simulink library "tqd"  (R2021b)
settings: Solver=VariableStepAuto  StartTime=0.0  StopTime=10.0  RelTol=1e-3
undefined symbols (not defined in the file or in its folder): ATQD_APSDecReq_X_kph, ATQD_APSDecReq_Y_mps2, ATQD_APSDecReqCMD_X_kph, ATQD_APSDecReqTs_X_pct, ATQD_APSDecTimeGain_X_Deg, ATQD_APSDecTimeGain_Y_s, ATQD_APSReqLowSpd_X_Deg, ATQD_AutoHoldReleaseBPS_X_Deg, ATQD_AWDLoadTrqnsGain_X_kg, ATQD_AWDLoadTrqnsGain_Y_pct, ATQD_BOSEnBPSPosn_X_kph, ATQD_BOSMap_X_rpm, ATQD_BOSMap_Y_pct, ATQD_CreepBaseTqD_X_kph, ATQD_CreepBaseTqD_Y_Deg, ATQD_CreepBaseTqR_X_kph, ATQD_CreepBaseTqR_Y_Deg, ATQD_CreepBPSDisPosn_X_Deg, ATQD_CreepBPSDisPosnR_X_Deg, ATQD_CreepBPSEnPosn_X_Deg, ATQD_CreepBPSEnPosnR_X_Deg, ATQD_CreepDeltaTq_X_kph, ATQD_CreepIterm_X_kph, ATQD_CreepIterm_Y_kph, ATQD_CreepItermMaxLimit_X_pct, ATQD_CreepPreloadTime_X_kph, ATQD_CreepPreloadTq_X_kph, ATQD_CreepPreloadTq_Y_s, ATQD_CreepProtTq_X_Deg, ATQD_CreepPterm_X_kph, ATQD_CreepPterm_Y_kph, ATQD_ECOTqMapD_X_rpm, ATQD_ECOTqMapD_Y_pct, ATQD_EOPDTqMapDCon_X_rpm, ATQD_EOPDTqMapDCon_Y_Deg, ATQD_EstInitVehWeight_X_c, ATQD_LHMRollGenMapD_X_rpm, ATQD_LHMRollGenMapD_Y_rpm, ATQD_LHMTqMapD_X_rpm, ATQD_LHMTqMapD_Y_pct, ATQD_NL1TqMapD_X_rpm, ATQD_NL1TqMapD_Y_pct, ATQD_NOPDTqMapDCon_X_rpm, ATQD_NOPDTqMapDCon_Y_Deg, ATQD_NRMRrEDUSpRat_X_rpm, ATQD_NRMRrEDUSpRat_Y_Nm, ATQD_OPDHoldDownRelDelay_X_Deg, ATQD_OPDHoldEnSpd_X_Deg, ATQD_OPDHoldRelDetTime_X_Deg, ATQD_OPDHoldReleaseTq_X_Deg, ATQD_OrigPedTqLowLim_X_Deg, ATQD_OrigPedTqLowLim_Y_pct, ATQD_PedalMapClimbUpLim_X_rpm, ATQD_PedalMapClimbUpLim_Y_Deg, ATQD_PreLoadTq_X_s, ATQD_RollGenMapEL1_X_rpm, ATQD_RollGenMapEL1_Y_rpm, ATQD_SL1TqMapD_X_rpm, ATQD_SL1TqMapD_Y_pct, ATQD_SlideRegenTqGain_X_Gps ... (+491)
libraries: hcu_lib x83, simulink x73, tqr x1
(part 15 of 19)

== system tqd/TQD/TorqueDemand/TorqueModule/DriverWhlTqDem/PedalMapWhlTq/NoLHM/ShiftD/LUT_D_Normal ==
  VTQD_TqTargetShaftSpd_rpm : Inport
  VTQD_ActAPSPosn_pct : Inport  Port=2
  VTQD_RegenMode_enum : Inport  Port=3
  VVMC_EstSlope_Deg : Inport  Port=4
  VTQD_APSReqTimer_s : Inport  Port=5
  VTQD_LowIdleAccPedal_flg : Inport  Port=6
  VTQD_OPDHoldEnRel_flg : Inport  Port=7
  VTQD_OPDHoldActRelTq_Nm : Inport  Port=8
  VTQD_VehActSpd_kph : Inport  Port=9
  VTQD_SlopeUp_flg : Inport  Port=10
  Action Port : ActionPort  ActionPortLabel=elseif(u2 ~= 0)
  Constant : Constant  Value=ENUM_REGENLEVEL_LV1
  Constant1 : Constant  Value=ENUM_REGENLEVEL_LV2
  Constant2 : Constant  Value=ENUM_REGENLEVEL_LV3
  Constant3 : Constant  Value=ENUM_REGENLEVEL_LV4
  Constant4 : Constant  Value=ENUM_REGENLEVEL_LV5
  Constant5 : Constant  Value=ENUM_REGENLEVEL_OPD
  Equal{1..6} (6 alike) : RelationalOperator  Operator===  OutDataTypeStr=boolean  RndMeth=Simplest
  If : If  NumInputs=6  IfExpression=u1 ~= 0  ElseIfExpressions=u2 ~= 0, u3 ~= 0, u4 ~= 0, u5 ~= 0, u6~=0
  MTQD_NL1TqMapD_Z_Nm : Lookup_n-D  BreakpointsForDimension1=ATQD_NL1TqMapD_Y_pct  BreakpointsForDimension2=ATQD_NL1TqMapD_X_rpm  Table=MTQD_NL1TqMapD_Z_Nm  ExtrapMethod=Clip  InternalRulePriority=Speed  RndMeth=Simplest  InputSameDT=on
      settings: InputPortMap=u0,u1
  MTQD_NL2TqMapD_Z_Nm : Lookup_n-D  BreakpointsForDimension1=ATQD_NL1TqMapD_Y_pct  BreakpointsForDimension2=ATQD_NL1TqMapD_X_rpm  Table=MTQD_NL2TqMapD_Z_Nm  ExtrapMethod=Clip  InternalRulePriority=Speed  RndMeth=Simplest  InputSameDT=on
      settings: InputPortMap=u0,u1
  MTQD_NL3TqMapD_Z_Nm : Lookup_n-D  BreakpointsForDimension1=ATQD_NL1TqMapD_Y_pct  BreakpointsForDimension2=ATQD_NL1TqMapD_X_rpm  Table=MTQD_NL3TqMapD_Z_Nm  ExtrapMethod=Clip  InternalRulePriority=Speed  RndMeth=Simplest  InputSameDT=on
      settings: InputPortMap=u0,u1
  MTQD_NL4TqMapD_Z_Nm1 : Lookup_n-D  BreakpointsForDimension1=ATQD_NL1TqMapD_Y_pct  BreakpointsForDimension2=ATQD_NL1TqMapD_X_rpm  Table=MTQD_NL4TqMapD_Z_Nm  ExtrapMethod=Clip  InternalRulePriority=Speed  RndMeth=Simplest  InputSameDT=on
      settings: InputPortMap=u0,u1
  MTQD_NL5TqMapD_Z_Nm1 : Lookup_n-D  BreakpointsForDimension1=ATQD_NL1TqMapD_Y_pct  BreakpointsForDimension2=ATQD_NL1TqMapD_X_rpm  Table=MTQD_NL5TqMapD_Z_Nm  ExtrapMethod=Clip  InternalRulePriority=Speed  RndMeth=Simplest  InputSameDT=on
      settings: InputPortMap=u0,u1
  MTQD_NOPDTqMapDCon_Z_Nm : Lookup_n-D  BreakpointsForDimension1=ATQD_NOPDTqMapDCon_Y_Deg  BreakpointsForDimension2=ATQD_NOPDTqMapDCon_X_rpm  Table=MTQD_NOPDTqMapDCon_Z_Nm  ExtrapMethod=Clip  InternalRulePriority=Speed  RndMeth=Simplest  InputSameDT=on
      settings: InputPortMap=u0,u1
  MTQD_NOPDTqMapD_Z_Nm1 : Lookup_n-D  BreakpointsForDimension1=ATQD_NL1TqMapD_Y_pct  BreakpointsForDimension2=ATQD_NL1TqMapD_X_rpm  Table=MTQD_NOPDTqMapD_Z_Nm  ExtrapMethod=Clip  InternalRulePriority=Speed  RndMeth=Simplest  InputSameDT=on
      settings: InputPortMap=u0,u1
  Merge : Merge  Inputs=7
  NRM_Invalid_TqMap1 : Subsystem  TreatAsAtomicUnit=on
  NRM_Lv1_TqMap : Subsystem  TreatAsAtomicUnit=on
  NRM_Lv2_TqMap : Subsystem  TreatAsAtomicUnit=on
  NRM_Lv3_TqMap : Subsystem  TreatAsAtomicUnit=on
  NRM_Lv4_TqMap : Subsystem  TreatAsAtomicUnit=on
  NRM_Lv5_TqMap : Subsystem  TreatAsAtomicUnit=on
  NRM_OnePedal_TqMap : Subsystem  TreatAsAtomicUnit=on
  VTQD_WhlTqNRMD_Nm : Outport
  wires:
  Equal6/1 -> If/6
  [VTQD_RegenMode_enum] -> Equal6/1
  Constant5/1 -> Equal6/2
  Equal5/1 -> If/5
  [VTQD_RegenMode_enum] -> Equal5/1
  Constant4/1 -> Equal5/2
  Equal4/1 -> If/4
  [VTQD_RegenMode_enum] -> Equal4/1
  Constant3/1 -> Equal4/2
  [VTQD_RegenMode_enum] -> Equal3/1
  Constant2/1 -> Equal3/2
  [VTQD_RegenMode_enum] -> Equal2/1
  Constant1/1 -> Equal2/2
  Constant/1 -> Equal1/2
  [VTQD_RegenMode_enum] -> Equal1/1
  [VTQD_NOPDTqMapD_Nm] -> NRM_OnePedal_TqMap/1(VTQD_NOPDTqMapDIn_Nm)
  If/6 -> NRM_OnePedal_TqMap/Action
  NRM_OnePedal_TqMap/1(VTQD_NOPDTqMapDOut_Nm) -> Merge/6
  [VTQD_NL5TqMapD_Nm] -> NRM_Lv5_TqMap/1(VTQD_NL5TqMapDIn_Nm)
  If/5 -> NRM_Lv5_TqMap/Action
  NRM_Lv5_TqMap/1(VTQD_NL5TqMapDOut_Nm) -> Merge/5
  NRM_Lv4_TqMap/1(VTQD_NL4TqMapDOut_Nm) -> Merge/4
  If/4 -> NRM_Lv4_TqMap/Action
  [VTQD_NL4TqMapD_Nm] -> NRM_Lv4_TqMap/1(VTQD_NL4TqMapDIn_Nm)
  [VTQD_NL3TqMapD_Nm] -> NRM_Lv3_TqMap/1(VTQD_NL3TqMapDIn_Nm)
  If/3 -> NRM_Lv3_TqMap/Action
  NRM_Lv3_TqMap/1(VTQD_NL3TqMapDOut_Nm) -> Merge/3
  [VTQD_NL2TqMapD_Nm] -> NRM_Lv2_TqMap/1(VTQD_NL2TqMapDIn_Nm)
  NRM_Lv2_TqMap/1(VTQD_NL2TqMapDOut_Nm) -> Merge/2
  If/2 -> NRM_Lv2_TqMap/Action
  NRM_Lv1_TqMap/1(VTQD_NL1TqMapDOut_Nm) -> Merge/1
  [VTQD_NL1TqMapD_Nm] -> NRM_Lv1_TqMap/1(VTQD_NL1TqMapDIn_Nm)
  Equal1/1 -> If/1
  Equal2/1 -> If/2
  If/1 -> NRM_Lv1_TqMap/Action
  Merge/1 -> VTQD_WhlTqNRMD_Nm/1
  Equal3/1 -> If/3
  [VTQD_TqTargetShaftSpd_rpm] -> MTQD_NOPDTqMapD_Z_Nm1/2
  [VTQD_ActAPSPosn_pct] -> MTQD_NOPDTqMapD_Z_Nm1/1
  [VTQD_TqTargetShaftSpd_rpm] -> MTQD_NL5TqMapD_Z_Nm1/2
  [VTQD_ActAPSPosn_pct] -> MTQD_NL5TqMapD_Z_Nm1/1
  [VTQD_TqTargetShaftSpd_rpm] -> MTQD_NL3TqMapD_Z_Nm/2
  [VTQD_ActAPSPosn_pct] -> MTQD_NL3TqMapD_Z_Nm/1
  [VTQD_TqTargetShaftSpd_rpm] -> MTQD_NL2TqMapD_Z_Nm/2
  [VTQD_ActAPSPosn_pct] -> MTQD_NL2TqMapD_Z_Nm/1
  MTQD_NL5TqMapD_Z_Nm1/1 -> [VTQD_NL5TqMapD_Nm]
  MTQD_NL4TqMapD_Z_Nm1/1 -> [VTQD_NL4TqMapD_Nm]
  [VTQD_TqTargetShaftSpd_rpm] -> MTQD_NL4TqMapD_Z_Nm1/2
  [VTQD_ActAPSPosn_pct] -> MTQD_NL4TqMapD_Z_Nm1/1
  MTQD_NOPDTqMapD_Z_Nm1/1 -> [VTQD_NOPDTqMapD_Nm]
  MTQD_NL3TqMapD_Z_Nm/1 -> [VTQD_NL3TqMapD_Nm]
  MTQD_NL2TqMapD_Z_Nm/1 -> [VTQD_NL2TqMapD_Nm]
  [VTQD_ActAPSPosn_pct] -> MTQD_NL1TqMapD_Z_Nm/1
  [VTQD_TqTargetShaftSpd_rpm] -> MTQD_NL1TqMapD_Z_Nm/2
  VTQD_RegenMode_enum/1 -> [VTQD_RegenMode_enum]
  VTQD_ActAPSPosn_pct/1 -> [VTQD_ActAPSPosn_pct]
  VTQD_TqTargetShaftSpd_rpm/1 -> [VTQD_TqTargetShaftSpd_rpm]
  MTQD_NL1TqMapD_Z_Nm/1 -> [VTQD_NL1TqMapD_Nm]
  [VTQD_NL1TqMapD_Nm] -> NRM_Invalid_TqMap1/1(VTQD_NL1TqMapDIn_Nm)
  If/7 -> NRM_Invalid_TqMap1/Action
  NRM_Invalid_TqMap1/1(VTQD_NL1TqMapDOut_Nm) -> Merge/7
  [VTQD_TqTargetShaftSpd_rpm] -> MTQD_NOPDTqMapDCon_Z_Nm/2
  [VVMC_EstSlope_Deg] -> MTQD_NOPDTqMapDCon_Z_Nm/1
  MTQD_NOPDTqMapDCon_Z_Nm/1 -> [VTQD_NOPDTqMapDCon_Nm]
  VVMC_EstSlope_Deg/1 -> [VVMC_EstSlope_Deg]
  [VTQD_NOPDTqMapDCon_Nm] -> NRM_OnePedal_TqMap/2(VTQD_NOPDTqMapDCon_Nm)
  [VTQD_APSReqTimer_s] -> NRM_OnePedal_TqMap/3(VTQD_APSReqTimer_s)
  VTQD_APSReqTimer_s/1 -> [VTQD_APSReqTimer_s]
  [VTQD_LowIdleAccPedal_flg] -> NRM_OnePedal_TqMap/4(VTQD_LowIdleAccPedal_flg)
  VTQD_LowIdleAccPedal_flg/1 -> [VTQD_LowIdleAccPedal_flg]
  VTQD_OPDHoldEnRel_flg/1 -> [VTQD_OPDHoldEnRel_flg]
  VTQD_OPDHoldActRelTq_Nm/1 -> [VTQD_OPDHoldActRelTq_Nm]
  VTQD_VehActSpd_kph/1 -> [VTQD_VehActSpd_kph]
  [VTQD_OPDHoldEnRel_flg] -> NRM_OnePedal_TqMap/5(VTQD_OPDHoldEnRel_flg)
  [VTQD_OPDHoldActRelTq_Nm] -> NRM_OnePedal_TqMap/6(VTQD_OPDHoldActRelTq_Nm)
  [VTQD_VehActSpd_kph] -> NRM_OnePedal_TqMap/7(VTQD_VehActSpd_kph)
  VTQD_SlopeUp_flg/1 -> [VTQD_SlopeUp_flg]
  [VTQD_SlopeUp_flg] -> NRM_OnePedal_TqMap/8(VTQD_SlopeUp_flg)

== system tqd/TQD/TorqueDemand/TorqueModule/DriverWhlTqDem/PedalMapWhlTq/NoLHM/ShiftD/LUT_D_SnowMode ==
  VTQD_TqTargetShaftSpd_rpm : Inport
  VTQD_ActAPSPosn_pct : Inport  Port=2
  VTQD_RegenMode_enum : Inport  Port=3
  VTQD_PreDecTqLowLim_Nm : Inport  Port=4
  Action Port : ActionPort  ActionPortLabel=if(u1 ~= 0)
  Constant1 : Constant  Value=ZERO_FLOAT
  Constant2 : Constant  Value=ENUM_REGENLEVEL_LV2
  Constant3 : Constant  Value=KTQD_PedalMapRDCUpLim_Nm
  Equal : RelationalOperator  Operator===  OutDataTypeStr=boolean  RndMeth=Simplest
  MTQD_SN1TqMapD_Z_Nm : Lookup_n-D  BreakpointsForDimension1=ATQD_SNTqMapD_Y_pct  BreakpointsForDimension2=ATQD_SNTqMapD_X_rpm  Table=MTQD_SNTqMapD_Z_Nm  ExtrapMethod=Clip  InternalRulePriority=Speed  RndMeth=Simplest  InputSameDT=on
      settings: InputPortMap=u0,u1
  Saturation Dynamic : simulink/Discontinuities/Saturation Dynamic  OutMin=[]  OutMax=[]  OutDataTypeStr=Inherit: Same as second input  OutDataType=fixdt(1, 16)  OutScaling=2^-10  DoSatur=off
  Switch : Switch  Criteria=u2 > Threshold
  VTQD_WhlTqSnowMode_Nm : Outport
  wires:
  VTQD_TqTargetShaftSpd_rpm/1 -> [VTQD_TqTargetShaftSpd_rpm]
  VTQD_ActAPSPosn_pct/1 -> [VTQD_ActAPSPosn_pct]
  VTQD_RegenMode_enum/1 -> [VTQD_RegenMode_enum]
  MTQD_SN1TqMapD_Z_Nm/1 -> [VTQD_SNTqMapD_Nm]  "VTQD_SNTqMapD_Nm"
  [VTQD_RegenMode_enum] -> Equal/1
  Equal/1 -> Switch/2
  Constant2/1 -> Equal/2
  [VTQD_ActAPSPosn_pct] -> MTQD_SN1TqMapD_Z_Nm/1
  [VTQD_TqTargetShaftSpd_rpm] -> MTQD_SN1TqMapD_Z_Nm/2
  Constant3/1 -> Saturation Dynamic/1
  VTQD_PreDecTqLowLim_Nm/1 -> [VTQD_PreDecTqLowLim_Nm]
  [VTQD_SNTqMapD_Nm] -> Saturation Dynamic/2
  Switch/1 -> Saturation Dynamic/3
  Saturation Dynamic/1 -> VTQD_WhlTqSnowMode_Nm/1
  Constant1/1 -> Switch/3
  [VTQD_PreDecTqLowLim_Nm] -> Switch/1

== system tqd/TQD/TorqueDemand/TorqueModule/DriverWhlTqDem/PedalMapWhlTq/NoLHM/ShiftD/LUT_D_Sport ==
  VTQD_TqTargetShaftSpd_rpm : Inport
  VTQD_ActAPSPosn_pct : Inport  Port=2
  VTQD_RegenMode_enum : Inport  Port=3
  VVMC_EstSlope_Deg : Inport  Port=4
  VTQD_APSReqTimer_s : Inport  Port=5
  VTQD_LowIdleAccPedal_flg : Inport  Port=6
  VTQD_OPDHoldEnRel_flg : Inport  Port=7
  VTQD_OPDHoldActRelTq_Nm : Inport  Port=8
  VTQD_VehActSpd_kph : Inport  Port=9
  VTQD_SlopeUp_flg : Inport  Port=10
  Action Port : ActionPort  ActionPortLabel=else
  Constant : Constant  Value=ENUM_REGENLEVEL_LV1
  Constant1 : Constant  Value=ENUM_REGENLEVEL_LV2
  Constant2 : Constant  Value=ENUM_REGENLEVEL_LV3
  Constant3 : Constant  Value=ENUM_REGENLEVEL_LV4
  Constant4 : Constant  Value=ENUM_REGENLEVEL_LV5
  Constant5 : Constant  Value=ENUM_REGENLEVEL_OPD
  Equal{1..6} (6 alike) : RelationalOperator  Operator===  OutDataTypeStr=boolean  RndMeth=Simplest
  If : If  NumInputs=6  IfExpression=u1 ~= 0  ElseIfExpressions=u2 ~= 0, u3 ~= 0, u4 ~= 0, u5 ~= 0, u6 ~= 0
  MTQD_SL1TqMapD_Z_Nm : Lookup_n-D  BreakpointsForDimension1=ATQD_SL1TqMapD_Y_pct  BreakpointsForDimension2=ATQD_SL1TqMapD_X_rpm  Table=MTQD_SL1TqMapD_Z_Nm  ExtrapMethod=Clip  InternalRulePriority=Speed  RndMeth=Simplest  InputSameDT=on
      settings: InputPortMap=u0,u1
  MTQD_SL2TqMapD_Z_Nm : Lookup_n-D  BreakpointsForDimension1=ATQD_SL1TqMapD_Y_pct  BreakpointsForDimension2=ATQD_SL1TqMapD_X_rpm  Table=MTQD_SL2TqMapD_Z_Nm  ExtrapMethod=Clip  InternalRulePriority=Speed  RndMeth=Simplest  InputSameDT=on
      settings: InputPortMap=u0,u1
  MTQD_SL3TqMapD_Z_Nm : Lookup_n-D  BreakpointsForDimension1=ATQD_SL1TqMapD_Y_pct  BreakpointsForDimension2=ATQD_SL1TqMapD_X_rpm  Table=MTQD_SL3TqMapD_Z_Nm  ExtrapMethod=Clip  InternalRulePriority=Speed  RndMeth=Simplest  InputSameDT=on
      settings: InputPortMap=u0,u1
  MTQD_SL4TqMapD_Z_Nm : Lookup_n-D  BreakpointsForDimension1=ATQD_SL1TqMapD_Y_pct  BreakpointsForDimension2=ATQD_SL1TqMapD_X_rpm  Table=MTQD_SL4TqMapD_Z_Nm  ExtrapMethod=Clip  InternalRulePriority=Speed  RndMeth=Simplest  InputSameDT=on
      settings: InputPortMap=u0,u1
  MTQD_SL5TqMapD_Z_Nm : Lookup_n-D  BreakpointsForDimension1=ATQD_SL1TqMapD_Y_pct  BreakpointsForDimension2=ATQD_SL1TqMapD_X_rpm  Table=MTQD_SL5TqMapD_Z_Nm  ExtrapMethod=Clip  InternalRulePriority=Speed  RndMeth=Simplest  InputSameDT=on
      settings: InputPortMap=u0,u1
  MTQD_SOPDTqMapDCon_Z_Nm : Lookup_n-D  BreakpointsForDimension1=ATQD_SOPDTqMapDCon_Y_Deg  BreakpointsForDimension2=ATQD_SOPDTqMapDCon_X_rpm  Table=MTQD_SOPDTqMapDCon_Z_Nm  ExtrapMethod=Clip  InternalRulePriority=Speed  RndMeth=Simplest  InputSameDT=on
      settings: InputPortMap=u0,u1
  MTQD_SOPDTqMapD_Z_Nm : Lookup_n-D  BreakpointsForDimension1=ATQD_SL1TqMapD_Y_pct  BreakpointsForDimension2=ATQD_SL1TqMapD_X_rpm  Table=MTQD_SOPDTqMapD_Z_Nm  ExtrapMethod=Clip  InternalRulePriority=Speed  RndMeth=Simplest  InputSameDT=on
      settings: InputPortMap=u0,u1
  Merge : Merge  Inputs=7
  Sport_Invalid_TqMap1 : Subsystem  TreatAsAtomicUnit=on
  Sport_Lv1_TqMap : Subsystem  TreatAsAtomicUnit=on
  Sport_Lv2_TqMap : Subsystem  TreatAsAtomicUnit=on
  Sport_Lv3_TqMap : Subsystem  TreatAsAtomicUnit=on
  Sport_Lv4_TqMap : Subsystem  TreatAsAtomicUnit=on
  Sport_Lv5_TqMap : Subsystem  TreatAsAtomicUnit=on
  Sport_OnePedal_TqMap : Subsystem  TreatAsAtomicUnit=on
  VTQD_WhlTqSPORTD_Nm : Outport
  wires:
  Equal6/1 -> If/6
  [VTQD_RegenMode_enum] -> Equal6/1
  Constant5/1 -> Equal6/2
  Equal5/1 -> If/5
  [VTQD_RegenMode_enum] -> Equal5/1
  Constant4/1 -> Equal5/2
  Equal4/1 -> If/4
  [VTQD_RegenMode_enum] -> Equal4/1
  Constant3/1 -> Equal4/2
  [VTQD_RegenMode_enum] -> Equal3/1
  Constant2/1 -> Equal3/2
  [VTQD_RegenMode_enum] -> Equal2/1
  Constant1/1 -> Equal2/2
  Constant/1 -> Equal1/2
  [VTQD_RegenMode_enum] -> Equal1/1
  [VTQD_SOPDTqMapD_Nm] -> Sport_OnePedal_TqMap/1(VTQD_SOPDTqMapDIn_Nm)
  If/6 -> Sport_OnePedal_TqMap/Action
  Sport_OnePedal_TqMap/1(VTQD_SOPDTqMapDOut_Nm) -> Merge/6
  [VTQD_SL5TqMapD_Nm] -> Sport_Lv5_TqMap/1(VTQD_SL5TqMapDIn_Nm)
  If/5 -> Sport_Lv5_TqMap/Action
  Sport_Lv5_TqMap/1(VTQD_SL5TqMapDOut_Nm) -> Merge/5
  Sport_Lv4_TqMap/1(VTQD_SL4TqMapDOut_Nm) -> Merge/4
  If/4 -> Sport_Lv4_TqMap/Action
  [VTQD_SL4TqMapD_Nm] -> Sport_Lv4_TqMap/1(VTQD_SL4TqMapDIn_Nm)
  [VTQD_SL3TqMapD_Nm] -> Sport_Lv3_TqMap/1(VTQD_SL3TqMapDIn_Nm)
  If/3 -> Sport_Lv3_TqMap/Action
  Sport_Lv3_TqMap/1(VTQD_SL3TqMapDOut_Nm) -> Merge/3
  [VTQD_SL2TqMapD_Nm] -> Sport_Lv2_TqMap/1(VTQD_SL2TqMapDIn_Nm)
  Sport_Lv2_TqMap/1(VTQD_SL2TqMapDOut_Nm) -> Merge/2
  If/2 -> Sport_Lv2_TqMap/Action
  Sport_Lv1_TqMap/1(VTQD_SL1TqMapDOut_Nm) -> Merge/1
  [VTQD_SL1TqMapD_Nm] -> Sport_Lv1_TqMap/1(VTQD_SL1TqMapDIn_Nm)
  Equal1/1 -> If/1
  Equal2/1 -> If/2
  If/1 -> Sport_Lv1_TqMap/Action
  Merge/1 -> VTQD_WhlTqSPORTD_Nm/1
  Equal3/1 -> If/3
  [VTQD_TqTargetShaftSpd_rpm] -> MTQD_SOPDTqMapD_Z_Nm/2
  [VTQD_ActAPSPosn_pct] -> MTQD_SOPDTqMapD_Z_Nm/1
  [VTQD_TqTargetShaftSpd_rpm] -> MTQD_SL5TqMapD_Z_Nm/2
  [VTQD_ActAPSPosn_pct] -> MTQD_SL5TqMapD_Z_Nm/1
  [VTQD_TqTargetShaftSpd_rpm] -> MTQD_SL3TqMapD_Z_Nm/2
  [VTQD_ActAPSPosn_pct] -> MTQD_SL3TqMapD_Z_Nm/1
  [VTQD_TqTargetShaftSpd_rpm] -> MTQD_SL2TqMapD_Z_Nm/2
  [VTQD_ActAPSPosn_pct] -> MTQD_SL2TqMapD_Z_Nm/1
  MTQD_SL5TqMapD_Z_Nm/1 -> [VTQD_SL5TqMapD_Nm]
  MTQD_SL4TqMapD_Z_Nm/1 -> [VTQD_SL4TqMapD_Nm]
  [VTQD_TqTargetShaftSpd_rpm] -> MTQD_SL4TqMapD_Z_Nm/2
  [VTQD_ActAPSPosn_pct] -> MTQD_SL4TqMapD_Z_Nm/1
  MTQD_SOPDTqMapD_Z_Nm/1 -> [VTQD_SOPDTqMapD_Nm]
  MTQD_SL3TqMapD_Z_Nm/1 -> [VTQD_SL3TqMapD_Nm]
  MTQD_SL2TqMapD_Z_Nm/1 -> [VTQD_SL2TqMapD_Nm]
  [VTQD_ActAPSPosn_pct] -> MTQD_SL1TqMapD_Z_Nm/1
  [VTQD_TqTargetShaftSpd_rpm] -> MTQD_SL1TqMapD_Z_Nm/2
  VTQD_RegenMode_enum/1 -> [VTQD_RegenMode_enum]
  VTQD_ActAPSPosn_pct/1 -> [VTQD_ActAPSPosn_pct]
  VTQD_TqTargetShaftSpd_rpm/1 -> [VTQD_TqTargetShaftSpd_rpm]
  MTQD_SL1TqMapD_Z_Nm/1 -> [VTQD_SL1TqMapD_Nm]
  [VTQD_SL1TqMapD_Nm] -> Sport_Invalid_TqMap1/1(VTQD_SL1TqMapDIn_Nm)
  If/7 -> Sport_Invalid_TqMap1/Action
  Sport_Invalid_TqMap1/1(VTQD_SL1TqMapDOut_Nm) -> Merge/7
  [VTQD_TqTargetShaftSpd_rpm] -> MTQD_SOPDTqMapDCon_Z_Nm/2
  [VVMC_EstSlope_Deg] -> MTQD_SOPDTqMapDCon_Z_Nm/1
  MTQD_SOPDTqMapDCon_Z_Nm/1 -> [VTQD_SOPDTqMapDCon_Nm]
  VVMC_EstSlope_Deg/1 -> [VVMC_EstSlope_Deg]
  VTQD_APSReqTimer_s/1 -> [VTQD_APSReqTimer_s]
  [VTQD_APSReqTimer_s] -> Sport_OnePedal_TqMap/3(VTQD_APSReqTimer_s)
  [VTQD_SOPDTqMapDCon_Nm] -> Sport_OnePedal_TqMap/2(VTQD_SOPDTqMapDCon_Nm)
  [VTQD_LowIdleAccPedal_flg] -> Sport_OnePedal_TqMap/4(VTQD_LowIdleAccPedal_flg)
  VTQD_LowIdleAccPedal_flg/1 -> [VTQD_LowIdleAccPedal_flg]
  VTQD_OPDHoldEnRel_flg/1 -> [VTQD_OPDHoldEnRel_flg]
  VTQD_VehActSpd_kph/1 -> [VTQD_VehActSpd_kph]
  VTQD_OPDHoldActRelTq_Nm/1 -> [VTQD_OPDHoldActRelTq_Nm]
  [VTQD_OPDHoldEnRel_flg] -> Sport_OnePedal_TqMap/5(VTQD_OPDHoldEnRel_flg)
  [VTQD_OPDHoldActRelTq_Nm] -> Sport_OnePedal_TqMap/6(VTQD_OPDHoldActRelTq_Nm)
  [VTQD_VehActSpd_kph] -> Sport_OnePedal_TqMap/7(VTQD_VehActSpd_kph)
  VTQD_SlopeUp_flg/1 -> [VTQD_SlopeUp_flg]
  [VTQD_SlopeUp_flg] -> Sport_OnePedal_TqMap/8(VTQD_SlopeUp_flg)

== system tqd/TQD/TorqueDemand/TorqueModule/DriverWhlTqDem/PedalMapWhlTq/NoLHM/ShiftD/LUT_D_ECO/ECO_Invalid_TqMap1 ==
  VTQD_RollRegenEnable_flg : Inport
  MTQD_RollGenMapEL1_Z_Nm : Inport  Port=2
  MTQD_ECOTqMapD_Z_Nm : Inport  Port=3
  Action Port : ActionPort
  Switch : Switch  Criteria=u2 ~= 0
  VTQD_EL1TqMapDOut_Nm : Outport
  wires:
  VTQD_RollRegenEnable_flg/1 -> Switch/2
  MTQD_RollGenMapEL1_Z_Nm/1 -> Switch/1
  MTQD_ECOTqMapD_Z_Nm/1 -> Switch/3
  Switch/1 -> VTQD_EL1TqMapDOut_Nm/1

== system tqd/TQD/TorqueDemand/TorqueModule/DriverWhlTqDem/PedalMapWhlTq/NoLHM/ShiftD/LUT_D_ECO/ECO_Lv1_TqMap ==
  VTQD_RollRegenEnable_flg : Inport
  MTQD_RollGenMapEL1_Z_Nm : Inport  Port=2
  MTQD_ECOTqMapD_Z_Nm : Inport  Port=3
  Action Port : ActionPort
  Switch : Switch  Criteria=u2 ~= 0
  VTQD_EL1TqMapDOut_Nm : Outport
  wires:
  Switch/1 -> VTQD_EL1TqMapDOut_Nm/1
  MTQD_ECOTqMapD_Z_Nm/1 -> Switch/3
  MTQD_RollGenMapEL1_Z_Nm/1 -> Switch/1
  VTQD_RollRegenEnable_flg/1 -> Switch/2

== system tqd/TQD/TorqueDemand/TorqueModule/DriverWhlTqDem/PedalMapWhlTq/NoLHM/ShiftD/LUT_D_ECO/ECO_Lv2_TqMap ==
  VTQD_EL2TqMapDIn_Nm : Inport
  Action Port : ActionPort
  VTQD_EL2TqMapDOut_Nm : Outport
  wires:
  VTQD_EL2TqMapDIn_Nm/1 -> VTQD_EL2TqMapDOut_Nm/1

== system tqd/TQD/TorqueDemand/TorqueModule/DriverWhlTqDem/PedalMapWhlTq/NoLHM/ShiftD/LUT_D_ECO/ECO_Lv3_TqMap ==
  VTQD_EL3TqMapDIn_Nm : Inport
  Action Port : ActionPort
  VTQD_EL3TqMapDOut_Nm : Outport
  wires:
  VTQD_EL3TqMapDIn_Nm/1 -> VTQD_EL3TqMapDOut_Nm/1

== system tqd/TQD/TorqueDemand/TorqueModule/DriverWhlTqDem/PedalMapWhlTq/NoLHM/ShiftD/LUT_D_ECO/ECO_Lv4_TqMap ==
  VTQD_EL4TqMapDIn_Nm : Inport
  Action Port : ActionPort
  VTQD_EL4TqMapDOut_Nm : Outport
  wires:
  VTQD_EL4TqMapDIn_Nm/1 -> VTQD_EL4TqMapDOut_Nm/1

== system tqd/TQD/TorqueDemand/TorqueModule/DriverWhlTqDem/PedalMapWhlTq/NoLHM/ShiftD/LUT_D_ECO/ECO_Lv5_TqMap ==
  VTQD_EL5TqMapDIn_Nm : Inport
  Action Port : ActionPort
  VTQD_EL5TqMapDOut_Nm : Outport
  wires:
  VTQD_EL5TqMapDIn_Nm/1 -> VTQD_EL5TqMapDOut_Nm/1

== system tqd/TQD/TorqueDemand/TorqueModule/DriverWhlTqDem/PedalMapWhlTq/NoLHM/ShiftD/LUT_D_ECO/ECO_OnePedal_TqMap ==
  VTQD_EOPDTqMapDIn_Nm : Inport
  VTQD_EOPDTqMapDCon_Nm : Inport  Port=2
  VTQD_APSReqTimer_s : Inport  Port=3
  VTQD_LowIdleAccPedal_flg : Inport  Port=4
  VTQD_OPDHoldEnRel_flg : Inport  Port=5
  VTQD_OPDHoldActRelTq_Nm : Inport  Port=6
  VTQD_VehActSpd_kph : Inport  Port=7
  VTQD_SlopeUp_flg : Inport  Port=8
  Action Port : ActionPort
  AND : Logic  AllPortsSameDT=off  OutDataTypeStr=boolean
  Add : Sum
  Constant1 : Constant  Value=ZERO_FLOAT
  Constant2 : Constant  Value=KTQD_OPDHTqDisComSpd_kph
  Constant9 : Constant  Value=KTQD_APSReqDelayTime_s
  Detect Increase : simulink/Logic and Bit Operations/Detect Increase  vinit=0.0  OutDataTypeStr=boolean
  Max : MinMax  Function=max  Inputs=2
  NOT : Logic  Operator=NOT  AllPortsSameDT=off  OutDataTypeStr=boolean
  OR : Logic  Operator=OR  Inputs=3  AllPortsSameDT=off  OutDataTypeStr=boolean
  Relational Operator : RelationalOperator  Operator=>  OutDataTypeStr=boolean  RndMeth=Simplest
  Relational Operator2 : RelationalOperator  OutDataTypeStr=boolean  RndMeth=Simplest
  SR_Latch : hcu_lib/Basic_Blocks/SR_Latch
  Switch : Switch  Criteria=u2 > Threshold
  Switch1 : Switch  Criteria=u2 > Threshold
  VTQD_EOPDTqMapDOut_Nm : Outport
  wires:
  Constant1/1 -> Switch/1
  VTQD_EOPDTqMapDCon_Nm/1 -> Switch/3
  VTQD_APSReqTimer_s/1 -> Relational Operator2/1
  Switch/1 -> Add/2
  Constant9/1 -> Relational Operator2/2
  VTQD_EOPDTqMapDIn_Nm/1 -> Add/1
  AND/1 -> Switch/2
  Relational Operator2/1 -> AND/1
  VTQD_LowIdleAccPedal_flg/1 -> [VTQD_LowIdleAccPedal_flg]
  [VTQD_LowIdleAccPedal_flg] -> AND/2
  Relational Operator/1 -> OR/2
  VTQD_OPDHoldActRelTq_Nm/1 -> Max/2
  [VTQD_LowIdleAccPedal_flg] -> OR/1
  Max/1 -> Switch1/1
  VTQD_OPDHoldEnRel_flg/1 -> Detect Increase/1
  VTQD_VehActSpd_kph/1 -> Relational Operator/1
  Detect Increase/1 -> SR_Latch/1
  Add/1 -> Max/1, Switch1/3  "VTQD_EOPDActTqMapD_Nm"
  OR/1 -> SR_Latch/2
  SR_Latch/1 -> Switch1/2
  Constant2/1 -> Relational Operator/2
  Switch1/1 -> VTQD_EOPDTqMapDOut_Nm/1
  NOT/1 -> OR/3
  VTQD_SlopeUp_flg/1 -> NOT/1

== system tqd/TQD/TorqueDemand/TorqueModule/DriverWhlTqDem/PedalMapWhlTq/NoLHM/ShiftD/LUT_D_Normal/NRM_Invalid_TqMap1 ==
  VTQD_NL1TqMapDIn_Nm : Inport
  Action Port : ActionPort
  VTQD_NL1TqMapDOut_Nm : Outport
  wires:
  VTQD_NL1TqMapDIn_Nm/1 -> VTQD_NL1TqMapDOut_Nm/1

== system tqd/TQD/TorqueDemand/TorqueModule/DriverWhlTqDem/PedalMapWhlTq/NoLHM/ShiftD/LUT_D_Normal/NRM_Lv1_TqMap ==
  VTQD_NL1TqMapDIn_Nm : Inport
  Action Port : ActionPort
  VTQD_NL1TqMapDOut_Nm : Outport
  wires:
  VTQD_NL1TqMapDIn_Nm/1 -> VTQD_NL1TqMapDOut_Nm/1

== system tqd/TQD/TorqueDemand/TorqueModule/DriverWhlTqDem/PedalMapWhlTq/NoLHM/ShiftD/LUT_D_Normal/NRM_Lv2_TqMap ==
  VTQD_NL2TqMapDIn_Nm : Inport
  Action Port : ActionPort
  VTQD_NL2TqMapDOut_Nm : Outport
  wires:
  VTQD_NL2TqMapDIn_Nm/1 -> VTQD_NL2TqMapDOut_Nm/1

== system tqd/TQD/TorqueDemand/TorqueModule/DriverWhlTqDem/PedalMapWhlTq/NoLHM/ShiftD/LUT_D_Normal/NRM_Lv3_TqMap ==
  VTQD_NL3TqMapDIn_Nm : Inport
  Action Port : ActionPort
  VTQD_NL3TqMapDOut_Nm : Outport
  wires:
  VTQD_NL3TqMapDIn_Nm/1 -> VTQD_NL3TqMapDOut_Nm/1

== system tqd/TQD/TorqueDemand/TorqueModule/DriverWhlTqDem/PedalMapWhlTq/NoLHM/ShiftD/LUT_D_Normal/NRM_Lv4_TqMap ==
  VTQD_NL4TqMapDIn_Nm : Inport
  Action Port : ActionPort
  VTQD_NL4TqMapDOut_Nm : Outport
  wires:
  VTQD_NL4TqMapDIn_Nm/1 -> VTQD_NL4TqMapDOut_Nm/1

== system tqd/TQD/TorqueDemand/TorqueModule/DriverWhlTqDem/PedalMapWhlTq/NoLHM/ShiftD/LUT_D_Normal/NRM_Lv5_TqMap ==
  VTQD_NL5TqMapDIn_Nm : Inport
  Action Port : ActionPort
  VTQD_NL5TqMapDOut_Nm : Outport
  wires:
  VTQD_NL5TqMapDIn_Nm/1 -> VTQD_NL5TqMapDOut_Nm/1

== system tqd/TQD/TorqueDemand/TorqueModule/DriverWhlTqDem/PedalMapWhlTq/NoLHM/ShiftD/LUT_D_Normal/NRM_OnePedal_TqMap ==
  VTQD_NOPDTqMapDIn_Nm : Inport
  VTQD_NOPDTqMapDCon_Nm : Inport  Port=2
  VTQD_APSReqTimer_s : Inport  Port=3
  VTQD_LowIdleAccPedal_flg : Inport  Port=4
  VTQD_OPDHoldEnRel_flg : Inport  Port=5
  VTQD_OPDHoldActRelTq_Nm : Inport  Port=6
  VTQD_VehActSpd_kph : Inport  Port=7
  VTQD_SlopeUp_flg : Inport  Port=8
  Action Port : ActionPort
  AND : Logic  AllPortsSameDT=off  OutDataTypeStr=boolean
  Add : Sum
  Constant1 : Constant  Value=ZERO_FLOAT
  Constant2 : Constant  Value=KTQD_OPDHTqDisComSpd_kph
  Constant9 : Constant  Value=KTQD_APSReqDelayTime_s
  Detect Increase : simulink/Logic and Bit Operations/Detect Increase  vinit=0.0  OutDataTypeStr=boolean
  Max : MinMax  Function=max  Inputs=2
  NOT : Logic  Operator=NOT  AllPortsSameDT=off  OutDataTypeStr=boolean
  OR : Logic  Operator=OR  Inputs=3  AllPortsSameDT=off  OutDataTypeStr=boolean
  Relational Operator : RelationalOperator  Operator=>  OutDataTypeStr=boolean  RndMeth=Simplest
  Relational Operator2 : RelationalOperator  OutDataTypeStr=boolean  RndMeth=Simplest
  SR_Latch : hcu_lib/Basic_Blocks/SR_Latch
  Switch : Switch  Criteria=u2 > Threshold
  Switch1 : Switch  Criteria=u2 > Threshold
  VTQD_NOPDTqMapDOut_Nm : Outport
  wires:
  Switch/1 -> Add/2
  VTQD_NOPDTqMapDIn_Nm/1 -> Add/1
  Constant9/1 -> Relational Operator2/2
  VTQD_APSReqTimer_s/1 -> Relational Operator2/1
  Constant1/1 -> Switch/1
  AND/1 -> Switch/2
  Relational Operator2/1 -> AND/1
  VTQD_LowIdleAccPedal_flg/1 -> [VTQD_LowIdleAccPedal_flg]
  [VTQD_LowIdleAccPedal_flg] -> AND/2
  VTQD_NOPDTqMapDCon_Nm/1 -> Switch/3
  VTQD_OPDHoldEnRel_flg/1 -> Detect Increase/1
  Detect Increase/1 -> SR_Latch/1
  SR_Latch/1 -> Switch1/2  "VTQD_OPDHoldRelPedTq_flg"
  Add/1 -> Max/1, Switch1/3  "VTQD_NOPDActTqMapD_Nm"
  Switch1/1 -> VTQD_NOPDTqMapDOut_Nm/1
  Max/1 -> Switch1/1
  VTQD_OPDHoldActRelTq_Nm/1 -> Max/2
  OR/1 -> SR_Latch/2
  [VTQD_LowIdleAccPedal_flg] -> OR/1
  Relational Operator/1 -> OR/2
  VTQD_VehActSpd_kph/1 -> Relational Operator/1
  Constant2/1 -> Relational Operator/2
  NOT/1 -> OR/3
  VTQD_SlopeUp_flg/1 -> NOT/1

== system tqd/TQD/TorqueDemand/TorqueModule/DriverWhlTqDem/PedalMapWhlTq/NoLHM/ShiftD/LUT_D_Sport/Sport_Invalid_TqMap1 ==
  VTQD_SL1TqMapDIn_Nm : Inport
  Action Port : ActionPort
  VTQD_SL1TqMapDOut_Nm : Outport
  wires:
  VTQD_SL1TqMapDIn_Nm/1 -> VTQD_SL1TqMapDOut_Nm/1

== system tqd/TQD/TorqueDemand/TorqueModule/DriverWhlTqDem/PedalMapWhlTq/NoLHM/ShiftD/LUT_D_Sport/Sport_Lv1_TqMap ==
  VTQD_SL1TqMapDIn_Nm : Inport
  Action Port : ActionPort
  VTQD_SL1TqMapDOut_Nm : Outport
  wires:
  VTQD_SL1TqMapDIn_Nm/1 -> VTQD_SL1TqMapDOut_Nm/1

== system tqd/TQD/TorqueDemand/TorqueModule/DriverWhlTqDem/PedalMapWhlTq/NoLHM/ShiftD/LUT_D_Sport/Sport_Lv2_TqMap ==
  VTQD_SL2TqMapDIn_Nm : Inport
  Action Port : ActionPort
  VTQD_SL2TqMapDOut_Nm : Outport
  wires:
  VTQD_SL2TqMapDIn_Nm/1 -> VTQD_SL2TqMapDOut_Nm/1

== system tqd/TQD/TorqueDemand/TorqueModule/DriverWhlTqDem/PedalMapWhlTq/NoLHM/ShiftD/LUT_D_Sport/Sport_Lv3_TqMap ==
  VTQD_SL3TqMapDIn_Nm : Inport
  Action Port : ActionPort
  VTQD_SL3TqMapDOut_Nm : Outport
  wires:
  VTQD_SL3TqMapDIn_Nm/1 -> VTQD_SL3TqMapDOut_Nm/1

== system tqd/TQD/TorqueDemand/TorqueModule/DriverWhlTqDem/PedalMapWhlTq/NoLHM/ShiftD/LUT_D_Sport/Sport_Lv4_TqMap ==
  VTQD_SL4TqMapDIn_Nm : Inport
  Action Port : ActionPort
  VTQD_SL4TqMapDOut_Nm : Outport
  wires:
  VTQD_SL4TqMapDIn_Nm/1 -> VTQD_SL4TqMapDOut_Nm/1

== system tqd/TQD/TorqueDemand/TorqueModule/DriverWhlTqDem/PedalMapWhlTq/NoLHM/ShiftD/LUT_D_Sport/Sport_Lv5_TqMap ==
  VTQD_SL5TqMapDIn_Nm : Inport
  Action Port : ActionPort
  VTQD_SL5TqMapDOut_Nm : Outport
  wires:
  VTQD_SL5TqMapDIn_Nm/1 -> VTQD_SL5TqMapDOut_Nm/1

== system tqd/TQD/TorqueDemand/TorqueModule/DriverWhlTqDem/PedalMapWhlTq/NoLHM/ShiftD/LUT_D_Sport/Sport_OnePedal_TqMap ==
  VTQD_SOPDTqMapDIn_Nm : Inport
  VTQD_SOPDTqMapDCon_Nm : Inport  Port=2
  VTQD_APSReqTimer_s : Inport  Port=3
  VTQD_LowIdleAccPedal_flg : Inport  Port=4
  VTQD_OPDHoldEnRel_flg : Inport  Port=5
  VTQD_OPDHoldActRelTq_Nm : Inport  Port=6
  VTQD_VehActSpd_kph : Inport  Port=7
  VTQD_SlopeUp_flg : Inport  Port=8
  Action Port : ActionPort
  AND : Logic  AllPortsSameDT=off  OutDataTypeStr=boolean
  Add : Sum
  Constant1 : Constant  Value=ZERO_FLOAT
  Constant2 : Constant  Value=KTQD_OPDHTqDisComSpd_kph
  Constant9 : Constant  Value=KTQD_APSReqDelayTime_s
  Detect Increase : simulink/Logic and Bit Operations/Detect Increase  vinit=0.0  OutDataTypeStr=boolean
  Max : MinMax  Function=max  Inputs=2
  NOT : Logic  Operator=NOT  AllPortsSameDT=off  OutDataTypeStr=boolean
  OR : Logic  Operator=OR  Inputs=3  AllPortsSameDT=off  OutDataTypeStr=boolean
  Relational Operator : RelationalOperator  Operator=>  OutDataTypeStr=boolean  RndMeth=Simplest
  Relational Operator2 : RelationalOperator  OutDataTypeStr=boolean  RndMeth=Simplest
  SR_Latch : hcu_lib/Basic_Blocks/SR_Latch
  Switch : Switch  Criteria=u2 > Threshold
  Switch1 : Switch  Criteria=u2 > Threshold
  VTQD_SOPDTqMapDOut_Nm : Outport
  wires:
  Constant1/1 -> Switch/1
  VTQD_SOPDTqMapDCon_Nm/1 -> Switch/3
  VTQD_APSReqTimer_s/1 -> Relational Operator2/1
  Switch/1 -> Add/2
  Constant9/1 -> Relational Operator2/2
  VTQD_SOPDTqMapDIn_Nm/1 -> Add/1
  AND/1 -> Switch/2
  Relational Operator2/1 -> AND/1
  Switch1/1 -> VTQD_SOPDTqMapDOut_Nm/1
  VTQD_LowIdleAccPedal_flg/1 -> [VTQD_LowIdleAccPedal_flg]
  [VTQD_LowIdleAccPedal_flg] -> AND/2
  NOT/1 -> OR/3
  Relational Operator/1 -> OR/2
  VTQD_OPDHoldActRelTq_Nm/1 -> Max/2
  [VTQD_LowIdleAccPedal_flg] -> OR/1
  Max/1 -> Switch1/1
  VTQD_OPDHoldEnRel_flg/1 -> Detect Increase/1
  VTQD_VehActSpd_kph/1 -> Relational Operator/1
  Detect Increase/1 -> SR_Latch/1
  Add/1 -> Max/1, Switch1/3  "VTQD_SOPDActTqMapD_Nm"
  OR/1 -> SR_Latch/2
  SR_Latch/1 -> Switch1/2
  Constant2/1 -> Relational Operator/2
  VTQD_SlopeUp_flg/1 -> NOT/1

== stateflow chart tqd/TQD/TorqueDemand/Signal_convert/SWC_Subsystem/Speed Setting Mode/ACC Speed Setting ON/ACCSetSpd_Chart_W ==
  state ACCSetSpeed_W
    (default) -> (junction 431) : {VTQD_ACCSetSpd_kph = ZERO_FLOAT;
        |  VTQD_ACCSavedSetSpd_kph = ZERO_FLOAT;
        |  VTQD_UpDownDetCount_sec = ZERO_FLOAT;
        |  VTQD_StandbyOvrdDetEnd_flg = FALSE;}
    ACCSetSpeed_W -> (junction 538) [order 3]
    (junction 538) -> (junction 552) [order 1] : [VTQD_DistanceUnit_flg == VINP_Distanceunit_flg || VTQD_ACCSavedSetSpd_kph <= ONE_FLOAT]
    (junction 552) -> (junction 431) : {VTQD_ACCSetSpd_kph = min(KTQD_ACCActiveMetSpdHi_raw32, VTQD_ACCSavedSetSpd_kph);
        |  VTQD_ACCSavedSetSpd_kph = VTQD_ACCSetSpd_kph;}
    (junction 538) -> (junction 540) [order 2]
    (junction 550) -> (junction 552)
    (junction 431) -> (junction 432) : {VSCP_ActiveDown_flg = FALSE;
        |  VTQD_ActiveUp_flg = FALSE;
        |  VTQD_UpDownTimeCount_sec = ZERO_FLOAT;}
    (junction 540) -> (junction 542) [order 1] : [VINP_Distanceunit_flg == TRUE]
    (junction 540) -> (junction 636) [order 2] : {VTQD_ACCSavedSetSpd_kph = (VTQD_ACCSavedSetSpd_kph * MPH2KPH)}
    (junction 542) -> (junction 599) : {VTQD_ACCSavedSetSpd_kph = (VTQD_ACCSavedSetSpd_kph * KPH2MPH)}
    (junction 432) -> (junction 530) [order 1] : [VINP_ADASACCSta_enum == ENUM_ADASACCSTA_STANDBY ||...
        |  VINP_ADASACCSta_enum == ENUM_ADASACCSTA_OVERRIDE]
    (junction 530) -> (junction 433) [order 1] : [VTQD_SWCSetDownSta_flg == TRUE ||...
        |  VTQD_SWCResUpSta_flg == TRUE]
    (junction 433) -> (junction 419) [order 1] : [VTQD_SWCSetDownSta_flg == TRUE &&...
        |  VTQD_StandbyOvrdDetEnd_flg == FALSE &&...
        |  VTQD_AllowSetSpd_flg == TRUE]
    (junction 432) -> (junction 403) [order 2]
    (junction 530) -> (junction 533) [order 2] : {VTQD_StandbyOvrdDetEnd_flg = FALSE;
        |  VTQD_ACCSetSpd_kph = VTQD_ACCSavedSetSpd_kph;
        |  VTQD_ACCSavedSetSpd_kph = VTQD_ACCSetSpd_kph;
        |  VTQD_DistanceUnit_flg = VINP_Distanceunit_flg;}
    (junction 433) -> (junction 490) [order 2]
    (junction 419) -> (junction 408) : {VTQD_UpDownDetCount_sec = VTQD_UpDownDetCount_sec + task_time_s;}
    (junction 599) -> (junction 602) [order 1] : [VTQD_ACCSavedSetSpd_kph < KTQD_ACCActiveMetSpdLoMPH_mph]
    (junction 636) -> (junction 623) [order 1] : [VTQD_ACCSavedSetSpd_kph < KTQD_ACCActiveMetSpdLo_kph]
    (junction 602) -> (junction 604) : {VTQD_ACCSavedSetSpd_kph = KTQD_ACCActiveMetSpdLoMPH_mph}
    (junction 636) -> (junction 633) [order 2]
    (junction 623) -> (junction 619) : {VTQD_ACCSavedSetSpd_kph = KTQD_ACCActiveMetSpdLo_kph}
    (junction 599) -> (junction 606) [order 2]
    (junction 604) -> (junction 606)
    (junction 619) -> (junction 633)
    (junction 606) -> (junction 613)
    (junction 633) -> (junction 630)
    (junction 630) -> (junction 625) [order 1] : [VTQD_ACCSavedSetSpd_kph > KTQD_ACCActiveMetSpdHi_kph]
    (junction 613) -> (junction 608) [order 1] : [VTQD_ACCSavedSetSpd_kph > KTQD_ACCActiveMetSpdHiMPH_mph]
    (junction 403) -> (junction 395) [order 1] : [(VTQD_SWCSetDownSta_flg == TRUE ||...
        |   VTQD_SWCResUpSta_flg == TRUE) &&...
        |  (VTQD_StandbyOvrdDetEnd_flg == TRUE ||...
        |   VTQD_HoldResDet_flg == TRUE)]
    (junction 490) -> (junction 492) [order 1] : [VINP_ADASACCSta_enum == ENUM_ADASACCSTA_STANDBY &&...
        |  VTQD_SWCResUpSta_flg == TRUE &&...
        |  VTQD_ACCSavedSetSpd_kph > ZERO_FLOAT]
    (junction 408) -> (junction 409) [order 1] : [VTQD_UpDownDetCount_sec > ZERO_FLOAT]
    (junction 409) -> (junction 405) [order 1] : [KTQD_ACCActiveMetSpdHi_raw32 >= VVMC_MeterIndSpeed_raw32 &&...
        |  VVMC_MeterIndSpeed_raw32 >= KTQD_ACCActiveMetSpdLo_raw32]
    (junction 630) -> (junction 632) [order 2]
    (junction 625) -> (junction 628) : {VTQD_ACCSavedSetSpd_kph = KTQD_ACCActiveMetSpdHi_kph}
    (junction 613) -> (junction 615) [order 2]
    (junction 608) -> (junction 612) : {VTQD_ACCSavedSetSpd_kph = KTQD_ACCActiveMetSpdHiMPH_mph}
    (junction 403) -> (junction 396) [order 2] : {VTQD_StandbyOvrdDetEnd_flg = FALSE;
        |  VTQD_HoldResDet_flg = FALSE;}
    (junction 395) -> (junction 399) : {VTQD_StandbyOvrdDetEnd_flg = TRUE;
        |  VTQD_HoldResDet_flg = TRUE;}
    (junction 490) -> (junction 496) [order 2]
    (junction 492) -> (junction 494) : {VTQD_StandbyOvrdDetEnd_flg = TRUE}
    (junction 408) -> (junction 436) [order 2] : {VTQD_ACCSetSpd_kph = VTQD_ACCSavedSetSpd_kph;
        |  VTQD_ACCSavedSetSpd_kph = VTQD_ACCSetSpd_kph;
        |  VTQD_DistanceUnit_flg = VINP_Distanceunit_flg;}
    (junction 409) -> (junction 410) [order 2]
    (junction 405) -> (junction 435) : {VTQD_ACCSetSpd_kph = VVMC_MeterIndSpeed_raw32;
        |  VTQD_ACCSavedSetSpd_kph = VTQD_ACCSetSpd_kph;
        |  VTQD_StandbyOvrdDetEnd_flg = TRUE;
        |  VTQD_UpDownDetCount_sec = ZERO_FLOAT;
        |  VTQD_DistanceUnit_flg = VINP_Distanceunit_flg;}
    (junction 628) -> (junction 632)
    (junction 612) -> (junction 615)
    (junction 632) -> (junction 547)
    (junction 615) -> (junction 544)
    (junction 547) -> (junction 544)
    (junction 544) -> (junction 550)
    (junction 494) -> (junction 496)
    (junction 410) -> (junction 429) [order 1] : [KTQD_ACCActiveMetSpdHi_raw32 < VVMC_MeterIndSpeed_raw32]
    (junction 496) -> (junction 407) : {VTQD_ACCSetSpd_kph = VTQD_ACCSavedSetSpd_kph;
        |  VTQD_ACCSavedSetSpd_kph = VTQD_ACCSetSpd_kph;
        |  VTQD_DistanceUnit_flg = VINP_Distanceunit_flg;}
    (junction 410) -> (junction 420) [order 2] : {VTQD_ACCSetSpd_kph = KTQD_ACCActiveMetSpdLo_raw32;
        |  VTQD_ACCSavedSetSpd_kph = VTQD_ACCSetSpd_kph;
        |  VTQD_StandbyOvrdDetEnd_flg = TRUE;
        |  VTQD_UpDownDetCount_sec = ZERO_FLOAT;
        |  VTQD_DistanceUnit_flg = VINP_Distanceunit_flg;}
    (junction 429) -> (junction 430) : {VTQD_ACCSetSpd_kph = KTQD_ACCActiveMetSpdHi_raw32;
        |  VTQD_ACCSavedSetSpd_kph = VTQD_ACCSetSpd_kph;
        |  VTQD_StandbyOvrdDetEnd_flg = TRUE;
        |  VTQD_UpDownDetCount_sec = ZERO_FLOAT;
        |  VTQD_DistanceUnit_flg = VINP_Distanceunit_flg;}
    (junction 399) -> (junction 396)
    (junction 396) -> (junction 438)
    (junction 438) -> (junction 417) [order 1] : [VINP_ADASACCSta_enum == ENUM_ADASACCSTA_ACTIVE]
    (junction 417) -> (junction 434) [order 1] : [VTQD_SWCSetDownSta_flg == TRUE &&...
        |  VTQD_StandbyOvrdDetEnd_flg == FALSE &&...
        |  VVMC_LVDAACCStatusInformation_flg == FALSE]
    (junction 438) -> (junction 427) [order 2]
    (junction 417) -> (junction 412) [order 2]
    (junction 434) -> (junction 411) : {VTQD_UpDownDetCount_sec = VTQD_UpDownDetCount_sec + task_time_s;}
    (junction 411) -> (junction 437) [order 1] : [VTQD_UpDownDetCount_sec > ZERO_FLOAT]
    (junction 411) -> (junction 406) [order 2] : {VTQD_ACCSetSpd_kph = VTQD_ACCSavedSetSpd_kph;
        |  VTQD_ACCSavedSetSpd_kph = VTQD_ACCSetSpd_kph;
        |  VTQD_DistanceUnit_flg = VINP_Distanceunit_flg;}
    (junction 437) -> (junction 428) : {VTQD_ACCSetSpd_kph = max(KTQD_ACCActiveMetSpdLo_raw32, VTQD_ACCSavedSetSpd_kph - ONE_FLOAT);
        |  VTQD_ACCSavedSetSpd_kph = VTQD_ACCSetSpd_kph;
        |  VSCP_ActiveDown_flg = TRUE;
        |  VTQD_UpDownDetCount_sec = ZERO_FLOAT;
        |  VTQD_UpDownTimeCount_sec = task_time_s;
        |  VTQD_DistanceUnit_flg = VINP_Distanceunit_flg;}
    (junction 427) -> (junction 404) [order 1] : [VINP_ADASACCSta_enum == ENUM_ADASACCSTA_OFF ||...
        |  VINP_ADASACCSta_enum == ENUM_ADASACCSTA_DISABLE||...
        |  VINP_ADASACCSta_enum == ENUM_ADASACCSTA_ERROR]
    (junction 412) -> (junction 510) [order 1] : [VTQD_SWCResUpSta_flg == TRUE]
    (junction 510) -> (junction 413) [order 1] : [VTQD_StandbyOvrdDetEnd_flg == FALSE &&...
        |  VVMC_LVDAACCStatusInformation_flg == FALSE &&...
        |  VTQD_HoldResDet_flg == FALSE]
    (junction 427) -> (junction 422) [order 2] : {VTQD_ACCSetSpd_kph = VTQD_ACCSavedSetSpd_kph;
        |  VTQD_ACCSavedSetSpd_kph = VTQD_ACCSetSpd_kph;
        |  VTQD_DistanceUnit_flg = VINP_Distanceunit_flg;}
    (junction 404) -> (junction 426) : {VTQD_ACCSetSpd_kph = ZERO_FLOAT;
        |  VTQD_ACCSavedSetSpd_kph = VTQD_ACCSetSpd_kph;
        |  VTQD_DistanceUnit_flg = VINP_Distanceunit_flg;}
    (junction 412) -> (junction 522) [order 2]
    (junction 510) -> (junction 512) [order 2]
    (junction 413) -> (junction 414) : {VTQD_UpDownDetCount_sec = VTQD_UpDownDetCount_sec + task_time_s;}
    (junction 512) -> (junction 514) [order 1] : [VTQD_StandbyOvrdDetEnd_flg == FALSE &&...
        |  VVMC_LVDAACCStatusInformation_flg != FALSE]
    (junction 414) -> (junction 415) [order 1] : [VTQD_UpDownDetCount_sec > ZERO_FLOAT]
    (junction 512) -> (junction 519) [order 2]
    (junction 514) -> (junction 516) : {VTQD_HoldResDet_flg = TRUE}
    (junction 414) -> (junction 418) [order 2] : {VTQD_ACCSetSpd_kph = VTQD_ACCSavedSetSpd_kph;
        |  VTQD_ACCSavedSetSpd_kph = VTQD_ACCSetSpd_kph;
        |  VTQD_DistanceUnit_flg = VINP_Distanceunit_flg;}
    (junction 415) -> (junction 421) : {VTQD_ACCSetSpd_kph = min(KTQD_ACCActiveMetSpdHi_raw32, VTQD_ACCSavedSetSpd_kph + ONE_FLOAT);
        |  VTQD_ACCSavedSetSpd_kph = VTQD_ACCSetSpd_kph;
        |  VTQD_ActiveUp_flg = TRUE;
        |  VTQD_UpDownDetCount_sec = ZERO_FLOAT;
        |  VTQD_UpDownTimeCount_sec = task_time_s;
        |  VTQD_DistanceUnit_flg = VINP_Distanceunit_flg;}
    (junction 519) -> (junction 522)
    (junction 516) -> (junction 519)
    (junction 522) -> (junction 416) : {VTQD_ACCSetSpd_kph = VTQD_ACCSavedSetSpd_kph;
        |  VTQD_ACCSavedSetSpd_kph = VTQD_ACCSetSpd_kph;
        |  VTQD_DistanceUnit_flg = VINP_Distanceunit_flg;}
    ACCSetSpeed_W -> (junction 568) [order 1] : [VSCP_ActiveDown_flg == TRUE &&...
        |  VINP_ADASACCSta_enum == ENUM_ADASACCSTA_ACTIVE &&...
        |  VTQD_SWCSetDownSta_flg == TRUE]
    (junction 568) -> (junction 556) [order 1] : [VTQD_DistanceUnit_flg == VINP_Distanceunit_flg]
    (junction 556) -> (junction 423)
    (junction 568) -> (junction 558) [order 2]
    (junction 560) -> (junction 556)
    (junction 423) -> (junction 424) : {VTQD_UpDownTimeCount_sec = VTQD_UpDownTimeCount_sec + task_time_s}
    (junction 558) -> (junction 566) [order 1] : [VINP_Distanceunit_flg == TRUE]
    (junction 558) -> (junction 571) [order 2] : {VTQD_ACCSavedSetSpd_kph = (VTQD_ACCSavedSetSpd_kph * MPH2KPH)}
    (junction 566) -> (junction 557) : {VTQD_ACCSavedSetSpd_kph = (VTQD_ACCSavedSetSpd_kph * KPH2MPH)}
    (junction 424) -> (junction 466) [order 1] : [VTQD_UpDownTimeCount_sec >= KTQD_SetSpdLongPLim_s]
    (junction 424) -> (junction 444) [order 2] : {VTQD_ACCSetSpd_kph = VTQD_ACCSavedSetSpd_kph;
        |  VTQD_ACCSavedSetSpd_kph = VTQD_ACCSetSpd_kph;
        |  VTQD_DistanceUnit_flg = VINP_Distanceunit_flg;}
    (junction 466) -> (junction 478) : {VTQD_ACCSetSpd_kph = max(KTQD_ACCActiveMetSpdLo_raw32, ceil(VTQD_ACCSavedSetSpd_kph / KTQD_SetSpdDeltaLong_kph - ONE_FLOAT) * KTQD_SetSpdDeltaLong_kph);
        |  VTQD_ACCSavedSetSpd_kph = VTQD_ACCSetSpd_kph;
        |  VTQD_UpDownTimeCount_sec = ZERO_FLOAT;
        |  VTQD_DistanceUnit_flg = VINP_Distanceunit_flg;}
    (junction 571) -> (junction 557)
    (junction 557) -> (junction 560)
    ACCSetSpeed_W -> (junction 585) [order 2] : [VTQD_ActiveUp_flg == TRUE &&...
        |  VINP_ADASACCSta_enum == ENUM_ADASACCSTA_ACTIVE &&...
        |  VTQD_SWCResUpSta_flg == TRUE]
    (junction 585) -> (junction 583) [order 1] : [VTQD_DistanceUnit_flg == VINP_Distanceunit_flg]
    (junction 583) -> (junction 479)
    (junction 585) -> (junction 584) [order 2]
    (junction 580) -> (junction 583)
    (junction 479) -> (junction 480) : {VTQD_UpDownTimeCount_sec = VTQD_UpDownTimeCount_sec + task_time_s}
    (junction 584) -> (junction 576) [order 1] : [VINP_Distanceunit_flg == TRUE]
    (junction 584) -> (junction 573) [order 2] : {VTQD_ACCSavedSetSpd_kph = (VTQD_ACCSavedSetSpd_kph * MPH2KPH)}
    (junction 576) -> (junction 582) : {VTQD_ACCSavedSetSpd_kph = (VTQD_ACCSavedSetSpd_kph * KPH2MPH)}
    (junction 480) -> (junction 463) [order 1] : [VTQD_UpDownTimeCount_sec >= KTQD_SetSpdLongPLim_s]
    (junction 480) -> (junction 455) [order 2] : {VTQD_ACCSetSpd_kph = VTQD_ACCSavedSetSpd_kph;
        |  VTQD_ACCSavedSetSpd_kph = VTQD_ACCSetSpd_kph;
        |  VTQD_DistanceUnit_flg = VINP_Distanceunit_flg;}
    (junction 463) -> (junction 461) : {VTQD_ACCSetSpd_kph = min(KTQD_ACCActiveMetSpdHi_raw32, floor(VTQD_ACCSavedSetSpd_kph / KTQD_SetSpdDeltaLong_kph + ONE_FLOAT) * KTQD_SetSpdDeltaLong_kph);
        |  VTQD_ACCSavedSetSpd_kph = VTQD_ACCSetSpd_kph;
        |  VTQD_UpDownTimeCount_sec = ZERO_FLOAT;
        |  VTQD_DistanceUnit_flg = VINP_Distanceunit_flg;}
    (junction 573) -> (junction 582)
    (junction 582) -> (junction 580)
  data: VINP_ADASACCSta_enum input uint8; VTQD_SWCResUpSta_flg input boolean; VTQD_SWCSetDownSta_flg input boolean; VVMC_MeterIndSpeed_raw32 input single; KTQD_ACCActiveMetSpdHi_raw32 input uint8; VINP_Distanceunit_flg input boolean; KTQD_ACCActiveMetSpdLo_raw32 input uint8; VTQD_ACCSetSpd_kph output single; KTQD_SetSpdDeltaLong_kph input uint8; VTQD_ACCSavedSetSpd_kph local single; ENUM_ADASACCSTA_STANDBY parameter uint8; ZERO_FLOAT parameter single; TRUE parameter boolean; ENUM_ADASACCSTA_ACTIVE parameter uint8; ONE_FLOAT parameter single; FALSE parameter boolean; VSCP_ActiveDown_flg local boolean; VTQD_UpDownTimeCount_sec local single; VTQD_ActiveUp_flg local boolean; KTQD_SetSpdLongPLim_s input single; VTQD_UpDownDetCount_sec local single; ENUM_ADASACCSTA_OVERRIDE parameter uint8; VTQD_StandbyOvrdDetEnd_flg local boolean; ENUM_ADASACCSTA_DISABLE parameter; ENUM_ADASACCSTA_OFF parameter; ENUM_ADASACCSTA_ERROR parameter; VVMC_LVDAACCStatusInformation_flg input; VTQD_HoldResDet_flg local boolean; VTQD_AllowSetSpd_flg input; task_time_s input; VTQD_DistanceUnit_flg local boolean; KPH2MPH parameter; MPH2KPH parameter; KTQD_ACCActiveMetSpdLo_kph parameter; KTQD_ACCActiveMetSpdLoMPH_mph parameter; KTQD_ACCActiveMetSpdHiMPH_mph parameter; KTQD_ACCActiveMetSpdHi_kph parameter
